simulink model "Rotatory"  (R2023b)
settings: Solver=VariableStepAuto  StartTime=0.0  StopTime=1.0  RelTol=1e-3
settings Model: Creator=Akaashdeep B  LastModifiedBy=Akaashdeep B

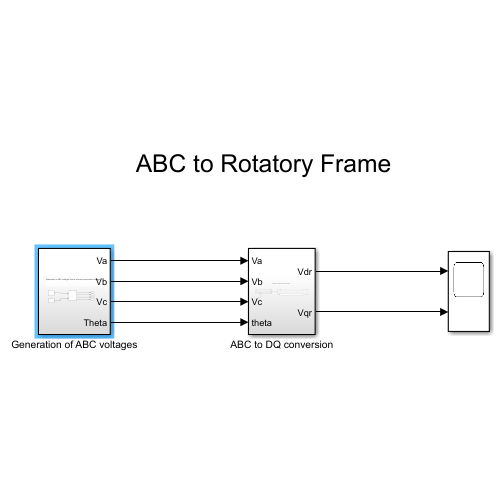
[thumbnail: Simulink's stored preview of the top-level diagram]
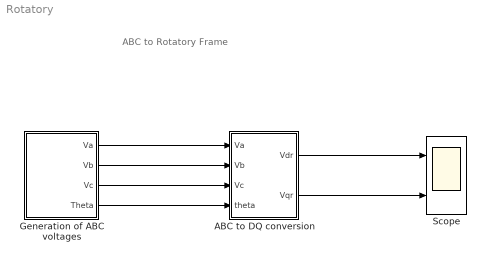
== system Rotatory ==
  note: ABC to Rotatory Frame
  ABC to DQ conversion : Subsystem
  Generation of ABC voltages : Subsystem
  Scope : Scope  NumInputPorts=2
  wires:
  ABC to DQ conversion/2(Vqr) -> Scope/2
  Generation of ABC voltages/4(Theta) -> ABC to DQ conversion/4(theta)
  Generation of ABC voltages/2(Vb) -> ABC to DQ conversion/2(Vb)
  Generation of ABC voltages/1(Va) -> ABC to DQ conversion/1(Va)
  Generation of ABC voltages/3(Vc) -> ABC to DQ conversion/3(Vc)
  ABC to DQ conversion/1(Vdr) -> Scope/1

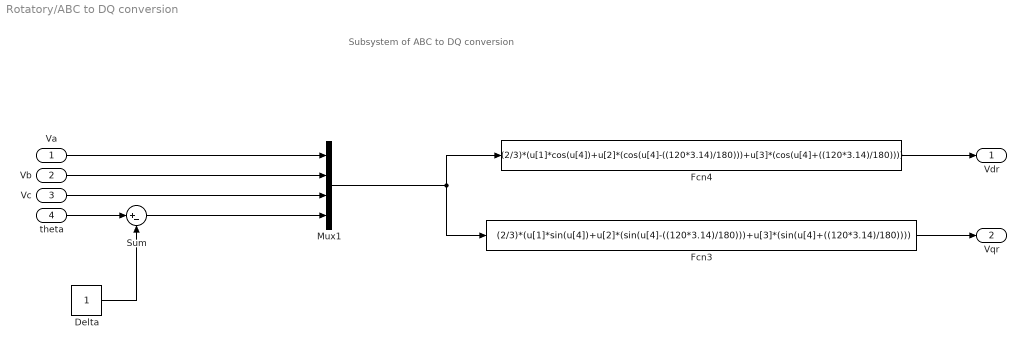
== system Rotatory/ABC to DQ conversion ==
  note: Subsystem of ABC to DQ conversion
  Va : Inport
  Vb : Inport  Port=2
  Vc : Inport  Port=3
  theta : Inport  Port=4
  Delta : Constant
  Fcn3 : Fcn  Expr=(2/3)*(u[1]*sin(u[4])+u[2]*(sin(u[4]-((120*3.14)/180)))+u[3]*(sin(u[4]+((120*3.14)/180))))
  Fcn4 : Fcn  Expr=(2/3)*(u[1]*cos(u[4])+u[2]*(cos(u[4]-((120*3.14)/180)))+u[3]*(cos(u[4]+((120*3.14)/180))))
  Mux1 : Mux
  Sum : Sum  Inputs=|+-
  Vdr : Outport
  Vqr : Outport  Port=2
  wires:
  Va/1 -> Mux1/1
  Vb/1 -> Mux1/2
  Mux1/1 -> Fcn4/1, Fcn3/1
  Fcn4/1 -> Vdr/1
  Vc/1 -> Mux1/3
  Fcn3/1 -> Vqr/1
  theta/1 -> Sum/1
  Delta/1 -> Sum/2
  Sum/1 -> Mux1/4

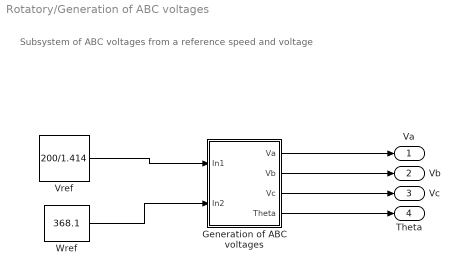
== system Rotatory/Generation of ABC voltages ==
  note: Subsystem of ABC voltages from a reference speed and voltage
  Generation of ABC voltages : Subsystem
  Vref : Constant  Value=200/1.414
  Wref : Constant  Value=368.1
  Va : Outport
  Vb : Outport  Port=2
  Vc : Outport  Port=3
  Theta : Outport  Port=4
  wires:
  Wref/1 -> Generation of ABC voltages/2(In2)
  Vref/1 -> Generation of ABC voltages/1(In1)
  Generation of ABC voltages/2(Vb) -> Vb/1
  Generation of ABC voltages/3(Vc) -> Vc/1
  Generation of ABC voltages/1(Va) -> Va/1
  Generation of ABC voltages/4(Theta) -> Theta/1

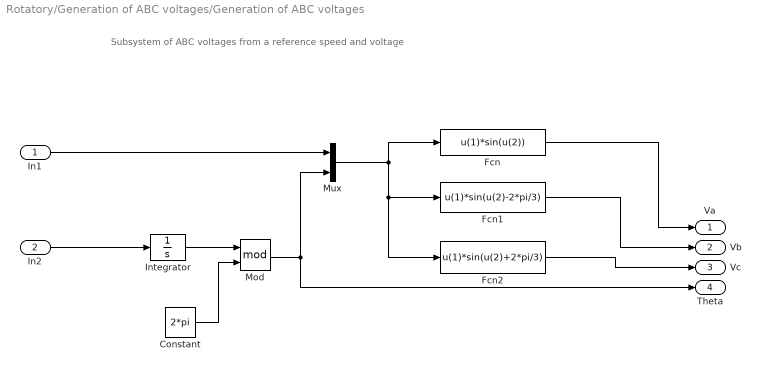
== system Rotatory/Generation of ABC voltages/Generation of ABC voltages ==
  note: Subsystem of ABC voltages from a reference speed and voltage
  In1 : Inport
  In2 : Inport  Port=2
  Constant : Constant  Value=2*pi
  Fcn : Fcn  Expr=u(1)*sin(u(2))
  Fcn1 : Fcn  Expr=u(1)*sin(u(2)-2*pi/3)
  Fcn2 : Fcn  Expr=u(1)*sin(u(2)+2*pi/3)
  Integrator : Integrator
  Mod : Math  Operator=mod
  Mux : Mux  Inputs=2
  Va : Outport
  Vb : Outport  Port=2
  Vc : Outport  Port=3
  Theta : Outport  Port=4
  wires:
  Mod/1 -> Theta/1, Mux/2
  Constant/1 -> Mod/2
  Mux/1 -> Fcn2/1, Fcn1/1, Fcn/1
  Fcn1/1 -> Vb/1
  Integrator/1 -> Mod/1
  Fcn/1 -> Va/1
  In1/1 -> Mux/1
  Fcn2/1 -> Vc/1
  In2/1 -> Integrator/1
